simulink model "mass_sping_damper"  (R2025b)
settings: Solver=VariableStepAuto  StartTime=0.0  StopTime=10.0  RelTol=1e-3
InitFcn:
  | mass_sping_damper_init
values from neighbouring files (symbols this model uses):
  msd_param = struct()    [mass_sping_damper_init.m]
undefined symbols (not defined in the file or in its folder): Kd, Ki, Kp
libraries: slpidlib x1
settings Model: Creator=Muhammed E. Hamamci  LastModifiedBy=hasanpul

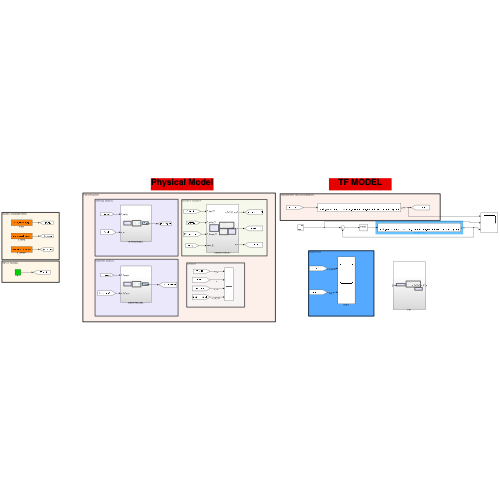
[thumbnail: Simulink's stored preview of the top-level diagram]
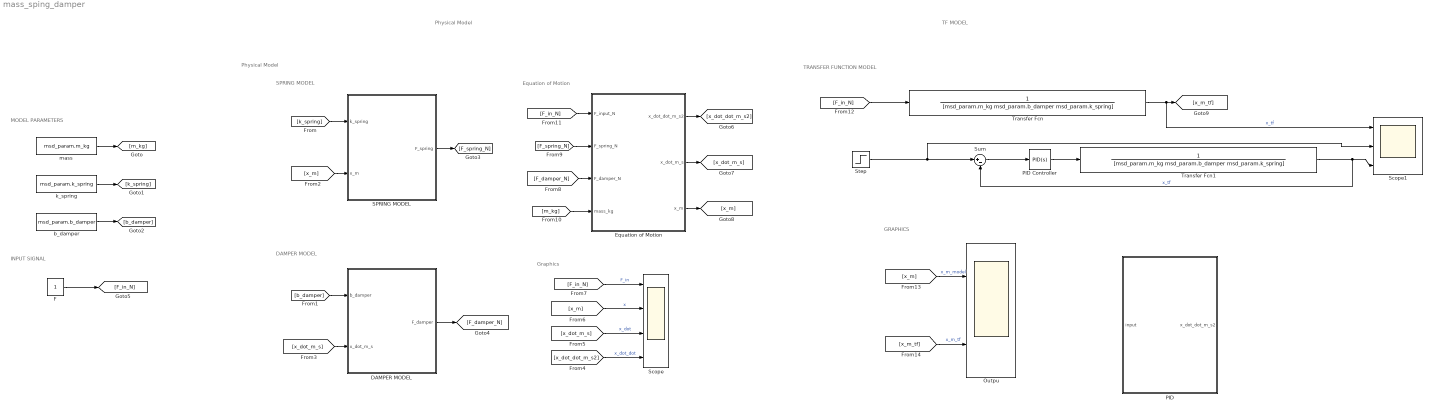
== system mass_sping_damper ==
  note: GRAPHICS
  note: TRANSFER FUNCTION MODEL
  note: Physical Model
  note: Physical Model
  note: Graphics
  note: Equation of Motion
  note: SPRING MODEL
  note: MODEL PARAMETERS
  note: DAMPER MODEL
  note: INPUT SIGNAL
  note: TF MODEL
  DAMPER MODEL : Subsystem
  Equation of Motion : Subsystem
  F : Constant
  Outpu : Scope  NumInputPorts=2
      settings: ActiveDisplayYMinimum=-1  ActiveDisplayYMaximum=1
  PID : Subsystem
  PID Controller : slpidlib/PID Controller  Controller=PID  Form=Parallel  TimeDomain=Continuous-time  UseExternalTs=off  SampleTime=-1  IntegratorMethod=Forward Euler  FilterMethod=Forward Euler  ControllerParametersSource=internal  P=350  I=300  UseKiTs=off  D=700  UseExternalDerivativeSource=off  N=482  UseFilter=on  TunerSelectOption=Transfer Function Based (PID Tuner App)  InitialConditionSource=internal  InitialConditionForIntegrator=0  InitialConditionForFilter=0  DifferentiatorICPrevScaledInput=0  ExternalReset=none  TrackingMode=off  Kt=1  LimitOutput=off  SatLimitsSource=internal  UpperSaturationLimit=inf  LowerSaturationLimit=-inf  LinearizeAsGain=on  AntiWindupMode=none  Kb=1  LimitIntegrator=off  UpperIntegratorSaturationLimit=inf  LowerIntegratorSaturationLimit=-inf  POutMin=[]  POutMax=[]  IOutMin=[]  IOutMax=[]  DOutMin=[]  DOutMax=[]  NOutMin=[]  NOutMax=[]  SumOutMin=[]  SumOutMax=[]  SaturationOutMin=[]  SaturationOutMax=[]  PParamMin=[]  PParamMax=[]  IParamMin=[]  IParamMax=[]  DParamMin=[]  DParamMax=[]  NParamMin=[]  NParamMax=[]  KbParamMin=[]  KbParamMax=[]  KtParamMin=[]  KtParamMax=[]  KbOutMin=[]  KbOutMax=[]  KtOutMin=[]  KtOutMax=[]  IntegratorOutMin=[]  IntegratorOutMax=[]  FilterOutMin=[]  FilterOutMax=[]  SumI1OutMin=[]  SumI1OutMax=[]  SumI2OutMin=[]  SumI2OutMax=[]  SumI3OutMin=[]  SumI3OutMax=[]  SumI4OutMin=[]  SumI4OutMax=[]  SumDOutMin=[]  SumDOutMax=[]  DifferentiatorOutMin=[]  DifferentiatorOutMax=[]  FilterDiffOutCoefMin=[]  FilterDiffOutCoefMax=[]  ReciprocalOutMin=[]  ReciprocalOutMax=[]  SumDenOutMin=[]  SumDenOutMax=[]  SumNumOutMin=[]  SumNumOutMax=[]  DivideOutMin=[]  DivideOutMax=[]  UdiffTsProdOutMin=[]  UdiffTsProdOutMax=[]  NTsProdOutMin=[]  NTsProdOutMax=[]  UintegralTsProdOutMin=[]  UintegralTsProdOutMax=[]  UngainTsProdOutMin=[]  UngainTsProdOutMax=[]  ClampingZeroOutDataTypeStr=Inherit: Inherit via back propagation  ClampingZeroOutMin=[]  ClampingZeroOutMax=[]  FilterDenConstantOutDataTypeStr=Inherit: Inherit via back propagation  FilterDenConstantOutMin=[]  FilterDenConstantOutMax=[]  PCopyOutDataTypeStr=Inherit: Inherit via back propagation  PCopyOutMin=[]  PCopyOutMax=[]  NCopyOutDataTypeStr=Inherit: Inherit via back propagation  NCopyOutMin=[]  NCopyOutMax=[]  IntegratorContinuousStateAttributes=''  IntegratorStateMustResolveToSignalObject=off  IntegratorRTWStateStorageClass=Auto  FilterContinuousStateAttributes=''  FilterStateMustResolveToSignalObject=off  FilterRTWStateStorageClass=Auto  ParallelPVariant=InternalParameters  IdealPVariant=Disabled  IVariant=InternalParameters  DVariant=InternalParameters  IntegratorVariant=Continuous  SatVariant=Disabled  AWVariant=Passthrough  PCopyVariant=Disabled  TRVariant=Disabled  FdbkBlocksVariant=Forward  IdealPFdbkVariant=Disabled  SatFdbkVariant=Disabled  DerivativeFilterVariant=ContFilter  NVariant=InternalParameters  NCopyVariant=Disabled  FilterICVariant=InternalICsFilter  IntegratorICVariant=InternalICs  ExternalResetVariant=Disabled  TRSumVariant=Passthrough  SumFdbkVariant=Disabled  SumVariant=Sum_PID  TsampFilterVariant=InternalTs  TsampNgainVariant=Passthrough  TsampIntegralVariant=Disabled_SignalSpec  ExternalSaturationOutDataTypeStr=Inherit: Same as second input  DerivativeSourceVariant=ErrorSignal  PreIntVariant=InternalPreInt
  SPRING MODEL : Subsystem
  Scope : Scope  NumInputPorts=4
      settings: ActiveDisplayYMinimum=-1  ActiveDisplayYMaximum=1
  Scope1 : Scope  NumInputPorts=3
      settings: ActiveDisplayString=3  ActiveDisplayYMinimum=-0.15199813815773885  ActiveDisplayYMaximum=1.36798324341965  DataLoggingVariableName=ScopeData2
  Step : Step  SampleTime=0
  Sum : Sum  Inputs=|+-
  Transfer Fcn : TransferFcn  Denominator=[msd_param.m_kg msd_param.b_damper msd_param.k_spring]
  Transfer Fcn1 : TransferFcn  Denominator=[msd_param.m_kg msd_param.b_damper msd_param.k_spring]
  b_damper : Constant  Value=msd_param.b_damper
  k_spring : Constant  Value=msd_param.k_spring
  mass : Constant  Value=msd_param.m_kg
  wires:
  mass/1 -> [m_kg]
  k_spring/1 -> [k_spring]
  b_damper/1 -> [b_damper]
  [k_spring] -> SPRING MODEL/1(k_spring)
  SPRING MODEL/1(F_spring) -> [F_spring_N]
  [b_damper] -> DAMPER MODEL/1(b_damper)
  DAMPER MODEL/1(F_damper) -> [F_damper_N]
  F/1 -> [F_in_N]
  Equation of Motion/1(x_dot_dot_m_s2) -> [x_dot_dot_m_s2]
  Equation of Motion/2(x_dot_m_s) -> [x_dot_m_s]
  Equation of Motion/3(x_m) -> [x_m]
  [x_m] -> SPRING MODEL/2(x_m)
  [x_dot_m_s] -> DAMPER MODEL/2(x_dot_m_s)
  [x_dot_dot_m_s2] -> Scope/4  "x_dot_dot"
  [x_dot_m_s] -> Scope/3  "x_dot"
  [x_m] -> Scope/2  "x"
  [F_in_N] -> Scope/1  "F_in"
  [F_damper_N] -> Equation of Motion/3(F_damper_N)
  [m_kg] -> Equation of Motion/4(mass_kg)
  [F_spring_N] -> Equation of Motion/2(F_spring_N)
  [F_in_N] -> Equation of Motion/1(F_input_N)
  [F_in_N] -> Transfer Fcn/1
  Transfer Fcn/1 -> Scope1/1, [x_m_tf]  "x_tf"
  [x_m] -> Outpu/1  "x_m_model"
  [x_m_tf] -> Outpu/2  "x_m_tf"
  Step/1 -> Scope1/2, Sum/1
  Sum/1 -> PID Controller/1
  Transfer Fcn1/1 -> Scope1/3, Sum/2  "x_tf"
  PID Controller/1 -> Transfer Fcn1/1

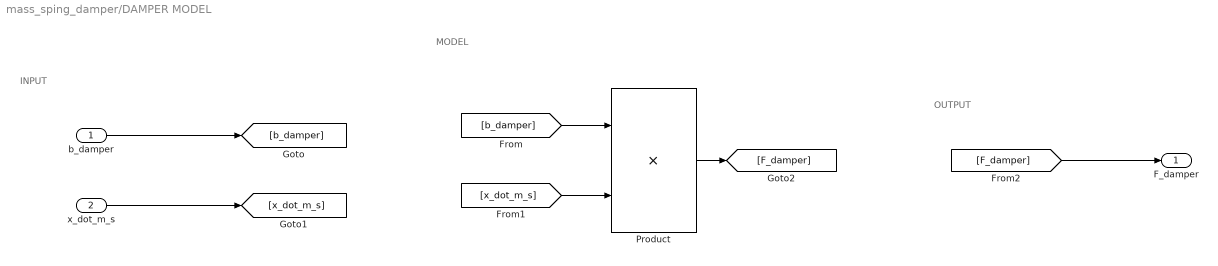
== system mass_sping_damper/DAMPER MODEL ==
  note: MODEL
  note: INPUT
  note: OUTPUT
  b_damper : Inport
  x_dot_m_s : Inport  Port=2
  Product : Product
  F_damper : Outport
  wires:
  x_dot_m_s/1 -> [x_dot_m_s]
  b_damper/1 -> [b_damper]
  [b_damper] -> Product/1
  [x_dot_m_s] -> Product/2
  [F_damper] -> F_damper/1
  Product/1 -> [F_damper]

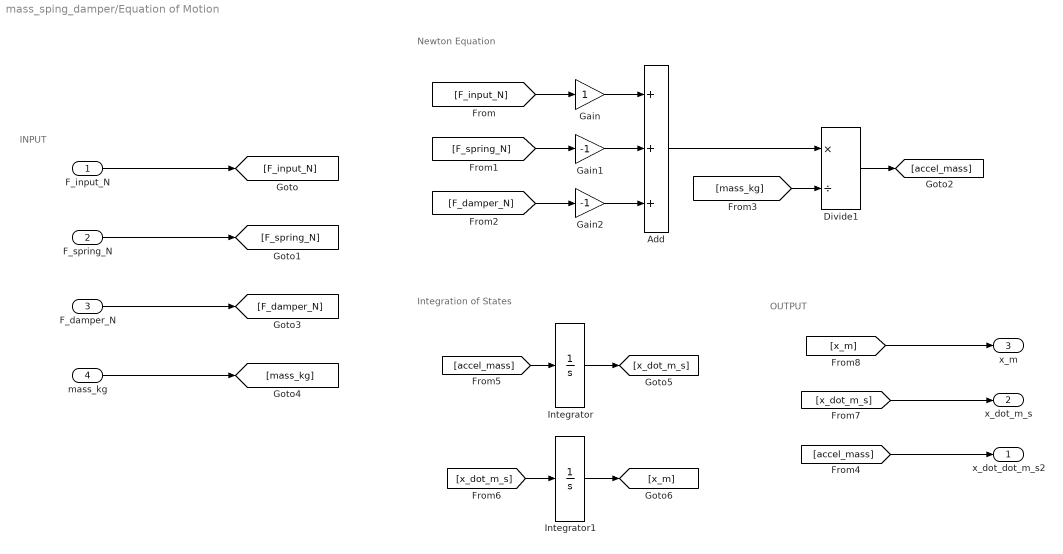
== system mass_sping_damper/Equation of Motion ==
  note: Newton Equation
  note: INPUT
  note: OUTPUT
  note: Integration of States
  F_input_N : Inport
  F_spring_N : Inport  Port=2
  F_damper_N : Inport  Port=3
  mass_kg : Inport  Port=4
  Add : Sum  Inputs=+++
  Divide1 : Product  Inputs=*/
  Gain : Gain
  Gain1 : Gain  Gain=-1
  Gain2 : Gain  Gain=-1
  Integrator : Integrator
  Integrator1 : Integrator
  x_dot_dot_m_s2 : Outport
  x_dot_m_s : Outport  Port=2
  x_m : Outport  Port=3
  wires:
  F_spring_N/1 -> [F_spring_N]
  F_input_N/1 -> [F_input_N]
  [accel_mass] -> x_dot_dot_m_s2/1
  F_damper_N/1 -> [F_damper_N]
  mass_kg/1 -> [mass_kg]
  [F_input_N] -> Gain/1
  [F_spring_N] -> Gain1/1
  [F_damper_N] -> Gain2/1
  Gain/1 -> Add/1
  Gain1/1 -> Add/2
  Gain2/1 -> Add/3
  Add/1 -> Divide1/1
  [mass_kg] -> Divide1/2
  Divide1/1 -> [accel_mass]
  [accel_mass] -> Integrator/1
  Integrator/1 -> [x_dot_m_s]
  [x_dot_m_s] -> Integrator1/1
  Integrator1/1 -> [x_m]
  [x_dot_m_s] -> x_dot_m_s/1
  [x_m] -> x_m/1

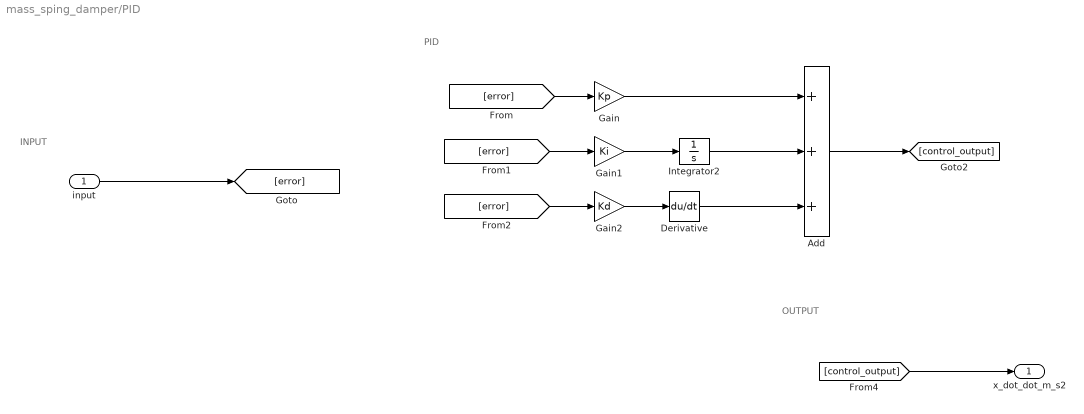
== system mass_sping_damper/PID ==
  note: PID
  note: INPUT
  note: OUTPUT
  input : Inport
  Add : Sum  Inputs=+++
  Derivative : Derivative
  Gain : Gain  Gain=Kp
  Gain1 : Gain  Gain=Ki
  Gain2 : Gain  Gain=Kd
  Integrator2 : Integrator
  x_dot_dot_m_s2 : Outport
  wires:
  input/1 -> [error]
  [control_output] -> x_dot_dot_m_s2/1
  [error] -> Gain/1
  Gain/1 -> Add/1
  Add/1 -> [control_output]
  [error] -> Gain1/1
  Gain1/1 -> Integrator2/1
  Integrator2/1 -> Add/2
  [error] -> Gain2/1
  Gain2/1 -> Derivative/1
  Derivative/1 -> Add/3

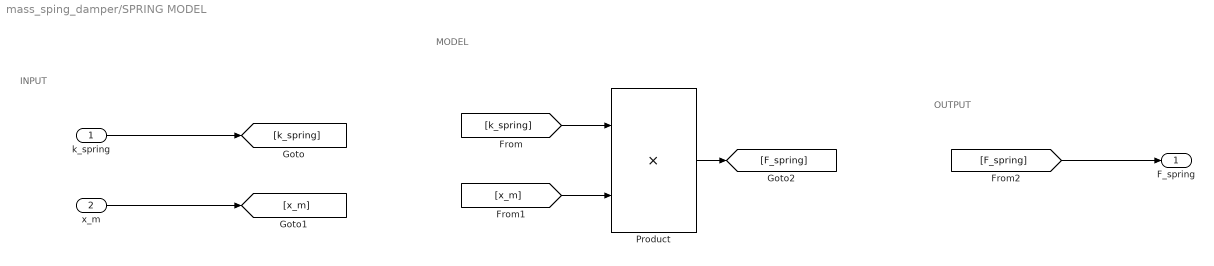
== system mass_sping_damper/SPRING MODEL ==
  note: MODEL
  note: INPUT
  note: OUTPUT
  k_spring : Inport
  x_m : Inport  Port=2
  Product : Product
  F_spring : Outport
  wires:
  x_m/1 -> [x_m]
  k_spring/1 -> [k_spring]
  [k_spring] -> Product/1
  [x_m] -> Product/2
  [F_spring] -> F_spring/1
  Product/1 -> [F_spring]
